simulink library "snn_champions_lib"  (R2026a)
settings: Solver=VariableStepAuto
(part 3 of 24)

== matlab function snn_champions_lib/Donatello_ACC_IIDM/SNN_ACC ==
  data: s input; accel output; v input; dv input; v_l input
function accel = SNN_ACC(s, v, dv, v_l)
%#codegen
% SP2 - campione Donatello + ACC-IIDM open-loop. ENTRAMBI in fixed -> HDL-ready.
%  Ingressi FIXED (>=20 bit frazionari); uscita accel (double). 1 cambio d'ingresso = 1
%  control-step = DT 0.1 s; ogni ingresso va tenuto >=341 campioni (time-mux).
  Tt = snn_types('fixed', 13);
  xn = local_normalize(s, v, dv, v_l, Tt);
  persistent pv xprev started acc
  if isempty(started)                % isempty(<persistent>) e' l'unica forma che il codegen
    pv = fi(zeros(5,1), 1, 21, 13);  % riconosce come prova di definizione: un test sul VALORE
    xprev = xn; started = true;      % fallirebbe con "undefined on some execution paths".
    Ta = acc_types('fixed'); acc = cast(0, 'like', Ta.out); go = true;
  else
    go = any(xn ~= xprev);           % edge-triggered: 1 campione = 1 inferenza
  end
  xprev = xn;
  [raw, valid] = snn_b2_fsm(xn, go);
  if valid
    pv = snn_decode_lut(raw, 64);
    % ⚠️ L'IIDM gira SOLO qui: una volta per control-step. A ogni clock vedrebbe Δv_l = 0 per
    %    340 campioni su 341 -> il filtro OU stimerebbe a_l ~ 0, in silenzio (spec §5).
    acc = acc_iidm_open(s, v, dv, v_l, pv(:), false, acc_types('fixed'));
  end
  accel = acc;                       % tenuto fino al control-step successivo
end

function xn = local_normalize(s, v, dv, v_l, T)
%LOCAL_NORMALIZE  fisico -> xn (fixed). Nel deployato la normalize gira in SW float e all'HDL
%  arriva gia' xn (HDL_PHASE §3.1); qui sta nel blocco per avere I/O fisico.
%  RECIPROCI a Q?.30 (NON Q?.20): verificato che con Q?.20 l'arrotondamento di xn devia di 1 LSB
%  dal path float ~1 volta su 25 step -> uno spike flippa -> i params divergono. Con Q?.30 e
%  ingressi con >=20 bit frazionari, xn e' IDENTICO al riferimento float (0 diff).
  invS   = fi(0.0066666666666666671, 1, 34, 30);
  invV   = fi(0.025000000000000001, 1, 34, 30);
  inv2DV = fi(0.025000000000000001, 1, 34, 30);
  invVL  = fi(0.025000000000000001, 1, 34, 30);
  DVc    = fi(20, 1, 24, 13);   % 24-13-1 = 10 bit interi: DV=20 ci sta
                                     % (con Q5.13/18bit saturerebbe a ~16 -> clamp sbagliato)
  d = dv;                            % clamp a +-DV. NB: d(:) = ... per NON cambiare il tipo di d
  if d >  DVc, d(:) =  DVc; end      %     (codegen: una variabile non puo' cambiare tipo, HDL_PHASE §9)
  if d < -DVc, d(:) = -DVc; end
  xn = cast(zeros(4,1), 'like', T.V);
  xn(1) = cast(s * invS, 'like', T.V);
  xn(2) = cast(v * invV, 'like', T.V);
  xn(3) = cast((d + DVc) * inv2DV, 'like', T.V);
  xn(4) = cast(v_l * invVL, 'like', T.V);
end

% ====================================================================================
% Funzioni locali INLINATE dai sorgenti veri (build_hdl_variants le legge a build-time).
% Le funzioni locali hanno precedenza sul path => il blocco e' SELF-CONTAINED.
% NON modificarle qui: si rigenerano con build_hdl_variants.
% ====================================================================================

function W = b2_rom_active() %#codegen
%B2_ROM_ACTIVE  Pesi del champion attivo (baked). GENERATO da gen_b2_rom('Donatello').
  W.fc = fi([1 1 -0.25 1;0.125 0.5 -0.0625 1;1 -1 1 0.125;1 0.125 0.5 -0.125;1 0.5 -0.0625 0.5;-0.0625 0.25 0 1;0 0.5 0.5 0.25;1 -0.25 2 -0.0625;1 0.125 -0.25 0.5;0.25 1 0.125 -0.25;0.25 -0.25 0.5 1;0.5 -0.5 0.5 0.25;1 0.25 -0.125 0.5;-1 1 0.25 0.5;1 0.5 1 -0.25;0.5 -0.25 0.5 0.0625;0.25 -0.25 1 -0.5;-0.5 -0.5 1 0.25;2 0 -0.25 0;-0.5 0.5 0.5 1;-0.125 -0.25 1 0;1 0.125 1 -0.5;-0.0625 1 0.5 0.125;1 1 -0.25 -0.125;2 0.5 0.5 -0.25;-0.125 0.5 0.25 -0.25;1 0.125 -0.0625 0.25;-0.5 -0.25 1 0.5;1 -0.125 0.125 0.5;1 -0.0625 0.5 0.25;1 0.5 1 0.125;0.125 0.25 0.5 0], 1, 16, 13);
  W.U = fi([0 0 -0.0625 -0.0625 -0.0625 0 0 0 -0.0625 0 0 0 0.0625 0 -0.125 0;-0.0625 0 -0.0625 0 0 0 0 0 0 0 -0.0625 0 0 0.0625 0 0;0.0625 -0.0625 -0.0625 0 -0.0625 -0.0625 0 0 0.0625 0 0.0625 0 0 0 0 0;0.0625 -0.0625 0 0 0 0 -0.0625 0 0 -0.0625 0.0625 -0.0625 0 -0.0625 0 -0.0625;0.0625 -0.0625 0 0 0 0 0.0625 0 0 0 0 -0.0625 0.0625 0 -0.0625 0;0 0.0625 0.0625 -0.0625 0.0625 0 0 0 0.0625 0.0625 0 0.0625 0 0 0 0;-0.0625 0.0625 0.0625 -0.0625 0 0 -0.0625 0.0625 0.0625 0.0625 0 0 -0.0625 0 0 0.0625;0 0 0.0625 0.0625 0 0 0 0 -0.0625 -0.0625 0 0 0 0 -0.0625 0;0 0 0 0 0.0625 -0.0625 0 0 -0.0625 -0.0625 -0.0625 0 0 0 0.0625 0;0 0 0 0 0.0625 0 0 0 0.0625 -0.0625 0 0.0625 0 0 0 0.0625;0 0 0 0 0 0 0 -0.0625 0 0 -0.0625 0 0 0 0 0.0625;0 0.0625 0 0.0625 0 0 0 0.0625 0 -0.0625 0 -0.0625 0.0625 0 0 0;-0.0625 0.0625 0 0 0 0 -0.0625 0 0.0625 0 -0.0625 0 0 0 0 0.125;0 0 0 0 0 0.0625 -0.0625 -0.0625 0 0.0625 0 0 0.0625 0.0625 0.0625 0;0.0625 0.0625 -0.0625 0 0 -0.0625 -0.0625 0 0 0 -0.0625 0 -0.0625 0 0 0;0.0625 0 0 0 -0.0625 -0.0625 -0.0625 0.0625 -0.0625 -0.0625 0 0.0625 0 0 0 0.0625;-0.0625 0 0 0 0.125 0.0625 -0.0625 -0.0625 0 0 0 0 -0.0625 0 -0.0625 0;0.0625 -0.0625 0 0.0625 0 -0.125 0 -0.0625 0 0 0.0625 -0.0625 0.0625 0 -0.0625 -0.0625;-0.0625 0 -0.0625 0.0625 -0.0625 0 -0.0625 0.0625 0.0625 -0.0625 0 0 -0.0625 0 0 -0.0625;0.0625 0.125 0 -0.0625 0 0 0 0 0.0625 0 0.0625 0.0625 0 0 -0.0625 0;0 -0.0625 0 0 -0.125 -0.0625 0 0.0625 -0.0625 -0.0625 0.0625 0 0.0625 -0.0625 -0.0625 -0.0625;0 0 0 0 -0.0625 0 0.0625 -0.0625 0 -0.0625 0.0625 0 0.0625 0 0 0;-0.0625 0.125 0 0 0 -0.0625 0 0 -0.0625 0.0625 0 0 0 0 0.0625 0;0 0 0 0 0 0 0 0 -0.0625 0 0.0625 0.125 0 0.0625 0 0.0625;0 -0.0625 0.0625 0 0 -0.0625 0 0 -0.0625 0 0 0.0625 0.0625 0 0 0;-0.0625 0 0 -0.125 0.0625 0.0625 0 0 0 0.0625 -0.0625 0.0625 -0.0625 0.0625 0.0625 0;0.0625 -0.0625 0 0 0 0 0.0625 0 -0.0625 0 0 0 0 0 0 0.0625;0 0 0 0.125 0 0 0 0.0625 -0.0625 0 0.0625 -0.0625 0 0.0625 0 0;0 0.0625 0.0625 0 0 0.0625 -0.0625 0 0 0.0625 0 0 -0.0625 0 0.0625 0.125;0 0.0625 0.0625 0.0625 0.0625 0.0625 0 0 0 0.0625 -0.0625 0.0625 -0.0625 0 0 0;0 0 0.0625 0 0 0.0625 -0.0625 -0.0625 0.0625 0.0625 -0.0625 0.125 0.0625 0 0 0;0 0 -0.0625 0.0625 0.0625 0 0 0.125 0 0.0625 0.0625 0.0625 0 -0.0625 0.0625 0], 1, 16, 13);
  W.Vr = fi([0 -0.125 -0.0625 -0.0625 0 0 -0.0625 -0.0625 0 -0.0625 -0.0625 0 0 0 -0.0625 -0.0625 0 0 0.0625 0 0 -0.125 0 0.0625 0 0 -0.0625 0 0 0 0 0;0.0625 0.0625 0 0 0 0 0.0625 0 0 0.0625 0.0625 0 0 0 0 0.0625 0 -0.0625 0 0.0625 0 0 0.0625 0 0.0625 0 0 0.125 -0.0625 0.125 0 0;0 0.0625 0 0.0625 0 0 -0.0625 0 0 0 0 0 0 0.0625 0 0 0.0625 0 0.0625 0 0 0.0625 0.0625 0 -0.0625 -0.0625 0 0 0 0.0625 0 0.0625;0 -0.0625 -0.0625 0 0 0 0 -0.0625 0 0 0.0625 0.0625 0 0 0 0.0625 0.0625 0 -0.0625 -0.0625 -0.0625 -0.0625 0.0625 0 0 0 0 0 0.0625 -0.0625 -0.0625 0;0 0 0.0625 0 -0.0625 0.0625 0.0625 0.0625 0 0 0.0625 0 0.0625 0.0625 0.0625 0 0.0625 0 0.0625 0 0.0625 0 0 0.0625 0.0625 0 0.125 0 0 0.0625 0.0625 0;0 0.0625 -0.125 0 0 0 0 0 0 -0.0625 -0.0625 0 0 0.0625 0.125 0.0625 0 0.0625 -0.0625 0.0625 0.0625 0 0.0625 -0.0625 0 -0.0625 0 0 0 0.0625 0 0;0 -0.0625 -0.0625 0 0 -0.0625 0 -0.0625 0 0 -0.0625 -0.0625 -0.0625 0.0625 -0.0625 0 0 -0.0625 0.0625 -0.125 -0.0625 0 -0.0625 -0.0625 -0.0625 0 0 -0.125 -0.0625 0 0 -0.0625;0 0 -0.0625 -0.0625 0.0625 0 -0.0625 0 -0.0625 0 0.0625 -0.0625 0.0625 0.0625 0.0625 0 0 0 0 -0.0625 0 -0.0625 0 0 0 0 -0.0625 -0.0625 0 0 0 0;-0.0625 0.0625 0 0.0625 0 0.0625 -0.0625 0 0.0625 0 0.0625 0 0 0.0625 0 0 0 0 0.0625 -0.0625 0.0625 0 0.0625 0 0 0.125 0.0625 0.0625 0.0625 0.0625 0 0;0.0625 0.0625 0 0.0625 0.0625 0.0625 0.0625 0.0625 0.0625 0 0.0625 0 0.0625 0.0625 0 -0.0625 0.0625 0 0.0625 0.0625 0 0.0625 0.0625 0 0.0625 0.0625 0 0 0 0 0 0;0 -0.0625 -0.0625 0 -0.0625 0 0 0 0 0 -0.0625 -0.125 -0.0625 -0.0625 0 -0.0625 -0.0625 0 0 -0.0625 -0.0625 0 0 0 0 -0.0625 0 -0.0625 0 0 -0.0625 0;0 0 0 0.0625 0 0 0.0625 0 0 0 0 0 0.0625 0 0 0.125 -0.0625 0 0.0625 0.0625 0 0 0.0625 0.0625 0 0.0625 0.0625 0 0 0 0 0;-0.0625 0 0 0 0.0625 0.0625 0 -0.0625 -0.0625 -0.0625 -0.0625 0 0 -0.0625 0 -0.0625 0 0 0 -0.0625 0 -0.0625 0 0 -0.0625 -0.0625 0 0 -0.0625 0 0.0625 0;0.0625 0 0 0.0625 0 0 0 -0.0625 0 0.0625 0 -0.0625 0 0.0625 0.0625 0 0.0625 0.0625 0 0.0625 0 0 0 0.0625 0.0625 0 0 0.125 0 0 0.0625 -0.0625;0.0625 0 0 0.0625 0 0.0625 0 0 0 0.0625 -0.0625 -0.0625 0 0.125 0 0 0 0 -0.0625 0 0.0625 0 0.0625 -0.0625 0.0625 0 0 0 0 0 0.0625 0;0 0 0 0.0625 0 0.0625 0 0.0625 0 0 0.0625 0.0625 0 0 0 0.0625 -0.0625 0 0.0625 0.0625 0.0625 0 0 0.0625 0.125 0 0 0 0 0 0.0625 0], 1, 19, 13);
  W.Wout = fi([-0.25 -0.125 -0.0625 -0.25 -0.25 0.25 0.25 -0.5 0.125 0.125 0.5 0.25 0.5 -0.125 0.25 0.25 -0.5 -0.25 0.0625 0.25 -0.25 0.0625 0 0.125 -0.25 0.25 0.25 -0.25 0 0 0.125 0.5;0.125 -0.125 0.25 -0.25 -0.125 0 -0.25 0 -0.25 0 0 0 -0.5 -0.5 0.125 0.25 -0.5 0.125 -0.25 0 0.25 0.25 -0.25 0.25 0.25 0 0.5 -0.25 -0.125 -0.25 0.0625 0.0625;0 -0.25 -0.25 0.125 -0.5 -0.0625 0 -0.125 0.125 0 0.25 -0.0625 -0.25 0.25 0.0625 -0.125 -0.25 0.125 -0.5 0.125 0.25 -0.5 -0.25 -0.25 0.25 0.25 0 0.5 -0.125 -0.5 0.125 0.125;0.5 0 0.25 0.25 0.25 -0.5 0.25 -0.25 0.5 0 -0.5 0.125 -0.0625 -0.5 -0.125 0.0625 0.25 -0.125 0.25 0.0625 0 0.0625 -0.25 -0.25 -0.125 -0.5 -0.25 0 -0.25 -0.125 -0.0625 -0.0625;-0.25 0 -0.0625 0.0625 0 -0.25 -0.125 -0.0625 -0.25 0 -0.0625 0.125 0.0625 0.25 -0.0625 -0.25 0.125 -0.25 -0.0625 -0.125 -0.25 -0.125 0.25 0.25 0.0625 0.25 -0.5 0.0625 0.25 0.25 -0.25 0.125], 1, 16, 13);
  W.bth = fi([1.4830578565597534;1.4914478063583374;1.4758200645446777;1.4738426208496094;1.4738566875457764;1.5251744985580444;1.5266332626342773;1.4767427444458008;1.4758551120758057;1.5250141620635986;1.5258395671844482;1.5129754543304443;1.5257152318954468;1.5249043703079224;1.5155367851257324;1.5183815956115723;1.5177655220031738;1.4894863367080688;1.4749715328216553;1.5253423452377319;1.4770052433013916;1.4827579259872437;1.5239431858062744;1.5230189561843872;1.4776254892349243;1.5125672817230225;1.5243701934814453;1.4934873580932617;1.5239229202270508;1.5202276706695557;1.5248651504516602;1.5149734020233154], 1, 19, 13);
  W.tj = fi([0.49987733364105225;0.49987733364105225;0.49987733364105225;0.49987733364105225;0.49987733364105225;0.49987733364105225;0.49987733364105225;0.49987733364105225;0.49987733364105225;0.49987733364105225;0.49987733364105225;0.49987733364105225;0.49987733364105225;0.49987733364105225;0.49987733364105225;0.49987733364105225;0.49987733364105225;0.49987733364105225;0.49987733364105225;0.49987733364105225;0.49987733364105225;0.49987733364105225;0.49987733364105225;0.49987733364105225;0.49987733364105225;0.49987733364105225;0.49987733364105225;0.49987733364105225;0.49987733364105225;0.49987733364105225;0.49987733364105225;0.49987733364105225], 1, 19, 13);
  W.delays = [3 5 1 2;2 4 4 4;2 4 0 4;5 0 5 5;1 2 2 2;4 1 4 2;0 4 0 1;0 1 0 1;2 2 1 3;1 2 5 2;0 5 1 2;0 5 3 1;2 0 0 4;2 2 3 4;4 4 5 0;4 5 0 2;0 4 4 3;5 5 4 2;4 5 4 2;3 0 3 1;3 2 0 4;0 4 2 0;5 4 5 2;4 4 3 3;5 3 4 5;2 2 3 1;3 3 5 3;1 3 0 3;1 0 3 2;2 3 4 4;2 4 5 0;1 2 4 0];
  W.sh = 3;
  W.invS = fi(0.0066666666666666671, 1, 24, 20);
  W.invV = fi(0.025000000000000001, 1, 24, 20);
  W.invVL = fi(0.025000000000000001, 1, 24, 20);
  W.inv2DV = fi(0.025000000000000001, 1, 24, 20);
  W.DV = fi(20, 1, 20, 13);
end


function T = snn_types(dt, nfrac)
%SNN_TYPES Prototipi di tipo per il core type-parametrizzato.
%  dt = 'double' (parita' vs golden) | 'fixed' (HDL, Qm.n).
%  nfrac (opz., default 5) = bit frazionari del path fixed; i bit INTERI restano
%  fissi (range invariato), varia solo la risoluzione -> per tarare i word-length
%  col ginocchio errore/risorse (run_fixed_sweep). nfrac=5 == config storica.
  if nargin < 2, nfrac = 5; end
  switch dt
    case 'double'
      z = double([]);
      T = struct('V', z, 'fatigue', z, 'acc', z, 'accw', z, 'raw', z, 'w', z);
    case 'fixed'
      f = nfrac;
      T = struct( ...
        'V',       fi([], true, 6 + f, f), ...    % Q5.f  (int 5)
        'fatigue', fi([], true, 4 + f, f), ...    % Q3.f  (int 3)
        'acc',     fi([], true, 6 + f, f), ...    % accumulatore I_input Q5.f (int 5: un tap di delay arriva a ~8)
        'accw',    fi([], true, 13 + f, f + 4), ...% accumulatore LARGO Q8.(f+4): +4 frac per shift po2 esatti
        'raw',     fi([], true, 8 + f, f), ...    % readout LI Q7.f (int 7)
        'w',       fi([], true, 3 + f, f));       % pesi po2 Q2.f (esatti per f>=5)
    otherwise
      error('snn_types:dt', 'dt deve essere ''double'' o ''fixed''');
  end
end


function [raw, valid] = snn_b2_fsm(xn, start) %#codegen
%SNN_B2_FSM  [B2] SNN Donatello time-multiplexato (1 neurone/clock) con hdl.RAM.
%  Mirror BIT-EXACT dell'aritmetica di snn_core, serializzato: V/fatigue in hdl.RAM,
%  pesi in ROM (coder.const), pipeline a 2 stadi per la latenza RAM (read->compute->write,
%  1 sola chiamata RAM/ciclo). Streaming: start=1 -> nuova control-step; valid=1 -> raw pronto.
  W = coder.const(b2_rom_active());
  T = snn_types('fixed', 13);
  hidden = 32; nt = 10; rnk = coder.const(size(W.U, 2)); out = 5; sh = W.sh;

  persistent Vram fatram xbuf xnreg t_lr t_lr_nxt V_LI wacc ...
             tickc rc written phase ...
             pR_valid pR_idx pCx_valid pCx_idx pCx_xsel pCx_Vread pCx_fat ...
             pCm_valid pCm_idx pCm_Iip pCm_recip pCm_Vread pCm_fat ...
             pCa_valid pCa_idx pCa_reci pCa_Ii pCa_Vread pCa_fat ...
             pC1_valid pC1_idx pC1_Ii pC1_reci pC1_Vread pC1_fat ...
             pC2i_valid pC2i_idx pC2i_Vi pC2i_eth pC2i_fat ...
             pC2a_valid pC2a_idx pC2a_nCV pC2a_sib pC2a_fat ...
             pC_valid pC_idx pC_V pC_fat rawreg inited
  if isempty(inited)
    Vram   = hdl.RAM('RAMType', 'Dual port');
    fatram = hdl.RAM('RAMType', 'Dual port');
    xbuf   = cast(zeros(4, 6), 'like', T.V);
    xnreg  = cast(zeros(4, 1), 'like', T.V);
    t_lr     = cast(zeros(rnk, 1), 'like', T.acc);
    t_lr_nxt = cast(zeros(rnk, 1), 'like', T.acc);
    V_LI = cast(zeros(out, 1), 'like', T.raw);
    wacc = cast(zeros(out, 1), 'like', T.raw);
    tickc = uint8(0); rc = uint8(0); written = uint8(0); phase = uint8(0);
    pR_valid = false; pR_idx = uint8(0);
    pCx_valid = false; pCx_idx = uint8(0);
    pCx_xsel = cast(zeros(4, 1), 'like', T.V);
    pCx_Vread = cast(0, 'like', T.V); pCx_fat = cast(0, 'like', T.fatigue);
    pCm_valid = false; pCm_idx = uint8(0);
    pCm_Iip = cast(zeros(4, 1), 'like', T.accw); pCm_recip = cast(zeros(rnk, 1), 'like', T.accw);
    pCm_Vread = cast(0, 'like', T.V); pCm_fat = cast(0, 'like', T.fatigue);
    pCa_valid = false; pCa_idx = uint8(0);
    pCa_reci = cast(zeros(rnk/4, 1), 'like', T.accw);   % rnk/4 somme parziali (dopo 2 livelli d'albero)
    pCa_Ii = cast(0, 'like', T.accw);
    pCa_Vread = cast(0, 'like', T.V); pCa_fat = cast(0, 'like', T.fatigue);
    pC1_valid = false; pC1_idx = uint8(0);
    pC1_Ii = cast(0, 'like', T.accw); pC1_reci = cast(0, 'like', T.accw);
    pC1_Vread = cast(0, 'like', T.V); pC1_fat = cast(0, 'like', T.fatigue);
    % [2d R8] prototipi dei tipi LARGHI di Vi/eth (l'addizione fixed li allarga oltre T.V): servono per
    % registrarli fra C2i (Vi/eth) e C2a (soglia/nC_V) senza conflitto di tipo in codegen.
    zV = cast(0, 'like', T.V); zA = cast(0, 'like', T.accw); zF = cast(0, 'like', T.fatigue);
    Vi0  = cast(zV - bitsra(zV, sh), 'like', T.V) + (zA + zA);
    eth0 = cast(zV, 'like', T.V) + cast(max(zF, zF), 'like', T.V);
    pC2i_valid = false; pC2i_idx = uint8(0);
    pC2i_Vi = cast(0, 'like', Vi0); pC2i_eth = cast(0, 'like', eth0);
    pC2i_fat = cast(0, 'like', T.fatigue);
    pC2a_valid = false; pC2a_idx = uint8(0);
    pC2a_nCV = cast(0, 'like', T.V); pC2a_sib = cast(0, 'like', T.V);
    pC2a_fat = cast(0, 'like', T.fatigue);
    pC_valid = false; pC_idx = uint8(0);
    pC_V = cast(0, 'like', T.V); pC_fat = cast(0, 'like', T.fatigue);
    rawreg = cast(zeros(out, 1), 'like', T.raw);
    inited = true;
  end

  valid = false;
  raw = rawreg;

  % ---------- helper x_buf: shift + inserimento xnreg (inizio tick) ----------
  % (fatto inline dove serve)

  if phase == uint8(0)
    % IDLE: su start latcha xn, fa lo shift del tick 0, avvia la pipeline
    if start
      xnreg = xn;
      xbuf(:, 2:6) = xbuf(:, 1:5); xbuf(:, 1) = xnreg;   % tick 0 shift+insert
      tickc = uint8(0); rc = uint8(0); written = uint8(0);
      wacc = cast(zeros(out, 1), 'like', T.raw);
      pR_valid = false; pC_valid = false;
      phase = uint8(1);
    end
    % passo RAM idle (mantiene coerenza)
    [~, ~] = Vram(cast(0,'like',T.V), uint8(0), false, uint8(0));
    [~, ~] = fatram(cast(0,'like',T.fatigue), uint8(0), false, uint8(0));
    return;
  end

  % ---------- FASE 1: RUN (pipeline 2-stadi, 1 chiamata RAM/ciclo) ----------
  % indirizzo di lettura per questo ciclo (neurone rc, se ancora da leggere)
  if rc < uint8(hidden), rdAddr = rc; else, rdAddr = uint8(0); end

  % UNA chiamata RAM: scrive il risultato dello stadio C (pC), legge rdAddr
  [~, Vread]   = Vram(pC_V,   pC_idx, pC_valid, rdAddr);
  [~, fatread] = fatram(pC_fat, pC_idx, pC_valid, rdAddr);
  if pC_valid
    written = written + uint8(1);
  end

  % --- STADIO Cx (mux xbuf: seleziona i 4 ingressi ritardati): dal neurone pR ---
  % [2d R9] separo il mux a indice variabile xbuf(j,col) dal DSP mult: Cx registra i 4 valori selezionati
  % (xsel), Cm fa solo i moltiplicatori dai valori registrati -> il mult (~4,6ns) resta l'unico op del suo path.
  nCx_valid = false; nCx_idx = uint8(0);
  nCx_xsel = cast(zeros(4, 1), 'like', T.V);
  nCx_Vread = cast(0, 'like', T.V); nCx_fat = cast(0, 'like', T.fatigue);
  if pR_valid
    i = double(pR_idx) + 1;
    for j = 1:4
      col = double(W.delays(i, j)) + 1;
      nCx_xsel(j) = xbuf(j, col);
    end
    nCx_Vread = Vread; nCx_fat = fatread;
    nCx_valid = true; nCx_idx = pR_idx;
  end

  % --- STADIO Cm (MAC: 16 prodotti reci + 4 prodotti Ii, REGISTRATI): dagli ingressi mux registrati pCx ---
  % [2d R6] isolo i moltiplicatori: Cm calcola e REGISTRA i prodotti (uscite DSP), Ca fa gli alberi dai
  % prodotti registrati -> il DSP mult (~4,6ns) esce dal path degli alberi (mappato sul registro P del DSP48).
  % Bit-exact: stessi prodotti, solo registrati.
  nCm_valid = false; nCm_idx = uint8(0);
  nCm_Iip = cast(zeros(4, 1), 'like', T.accw);
  nCm_recip = cast(zeros(rnk, 1), 'like', T.accw);
  nCm_Vread = cast(0, 'like', T.V); nCm_fat = cast(0, 'like', T.fatigue);
  if pCx_valid
    i = double(pCx_idx) + 1;
    for j = 1:4
      nCm_Iip(j) = cast(cast(W.fc(i, j), 'like', T.w) * pCx_xsel(j), 'like', T.accw);
    end
    for r = 1:rnk
      nCm_recip(r) = cast(cast(W.U(i, r), 'like', T.w) * t_lr(r), 'like', T.accw);
    end
    nCm_Vread = pCx_Vread; nCm_fat = pCx_fat;
    nCm_valid = true; nCm_idx = pCx_idx;
  end

  % --- STADIO Ca (alberi: Ii 4->1, reci L1-L2 16->4): dai prodotti registrati pCm ---
  kmid = coder.const(rnk / 4);                    % rnk=16 -> 4 parziali dopo 2 livelli
  nCa_valid = false; nCa_idx = uint8(0);
  nCa_reci = cast(zeros(kmid, 1), 'like', T.accw);
  nCa_Ii = cast(0, 'like', T.accw);
  nCa_Vread = cast(0, 'like', T.V); nCa_fat = cast(0, 'like', T.fatigue);
  if pCm_valid
    % Ii ad albero (4->2->1) dai prodotti registrati
    Ii_p = pCm_Iip;
    Ii_p(1) = cast(Ii_p(1) + Ii_p(2), 'like', T.accw);
    Ii_p(2) = cast(Ii_p(3) + Ii_p(4), 'like', T.accw);
    nCa_Ii  = cast(Ii_p(1) + Ii_p(2), 'like', T.accw);
    % reci: primi 2 livelli d'albero (16->4) dai prodotti registrati
    reci_p = pCm_recip;
    lvsz_a = coder.const(round(rnk ./ 2 .^ (1:2)));   % rnk=16 -> [8 4]
    for lev = 1:2
      for q = 1:lvsz_a(lev)
        reci_p(q) = cast(reci_p(2*q - 1) + reci_p(2*q), 'like', T.accw);
      end
    end
    nCa_reci = reci_p(1:kmid);            % rnk/4 somme parziali (T.accw)
    nCa_Vread = pCm_Vread; nCa_fat = pCm_fat;
    nCa_valid = true; nCa_idx = pCm_idx;
  end

  % --- STADIO C1 (SECONDA meta' dell'albero reci): dal registro pCa ---
  nC1_valid = false; nC1_idx = uint8(0);
  nC1_Ii = cast(0, 'like', T.accw); nC1_reci = cast(0, 'like', T.accw);
  nC1_Vread = cast(0, 'like', T.V); nC1_fat = cast(0, 'like', T.fatigue);
  if pCa_valid
    reci_p2 = pCa_reci;                  % kmid parziali
    lvsz_b = coder.const(round(kmid ./ 2 .^ (1:log2(kmid))));   % kmid=4 -> [2 1]
    for lev = 1:numel(lvsz_b)
      for q = 1:lvsz_b(lev)
        reci_p2(q) = cast(reci_p2(2*q - 1) + reci_p2(2*q), 'like', T.accw);
      end
    end
    nC1_reci = reci_p2(1);
    nC1_Ii = pCa_Ii; nC1_Vread = pCa_Vread; nC1_fat = pCa_fat;   % Vi/soglia -> C2 (tipi larghi restano locali)
    nC1_valid = true; nC1_idx = pCa_idx;
  end

  % --- STADIO C2i (calcola Vi ed eth, tipi larghi 28-bit): dal registro pC1 ---
  % [2d R8] separo Vi/eth (catena di add 28-bit, era il collo in C2a-R7) dalla soglia/nC_V: C2i li produce
  % e REGISTRA (tipi larghi via prototipo Vi0/eth0 in init; init nel corpo via 'like' pC2i_*). Bit-exact.
  nC2i_valid = false; nC2i_idx = uint8(0);
  nC2i_Vi = cast(0, 'like', pC2i_Vi); nC2i_eth = cast(0, 'like', pC2i_eth);
  nC2i_fat = cast(0, 'like', T.fatigue);
  if pC1_valid
    i2 = double(pC1_idx) + 1;
    nC2i_Vi  = cast(pC1_Vread - bitsra(pC1_Vread, sh), 'like', T.V) + (pC1_Ii + pC1_reci);
    nC2i_eth = cast(W.bth(i2), 'like', T.V) + cast(max(pC1_fat, cast(0,'like',T.fatigue)), 'like', T.V);
    nC2i_fat = pC1_fat;
    nC2i_valid = true; nC2i_idx = pC1_idx;
  end

  % --- STADIO C2a (soglia + nC_V + accumulo readout): dal registro pC2i ---
  nC2a_valid = false; nC2a_idx = uint8(0);
  nC2a_nCV = cast(0, 'like', T.V); nC2a_sib = cast(0, 'like', T.V);
  nC2a_fat = cast(0, 'like', T.fatigue);
  if pC2i_valid
    i2  = double(pC2i_idx) + 1;
    si  = pC2i_Vi >= pC2i_eth;
    sib = cast(si, 'like', T.V);
    nC2a_nCV = cast(pC2i_Vi - sib * pC2i_eth, 'like', T.V);
    nC2a_sib = sib; nC2a_fat = pC2i_fat;
    nC2a_valid = true; nC2a_idx = pC2i_idx;
    if si
      for o = 1:out
        wacc(o) = cast(wacc(o) + W.Wout(o, i2), 'like', T.raw);
      end
      for r = 1:rnk
        t_lr_nxt(r) = cast(t_lr_nxt(r) + cast(W.Vr(r, i2), 'like', T.acc), 'like', T.acc);
      end
    end
  end

  % --- STADIO C2b (nC_fat = leaky(fat) + sib*tj): dal registro pC2a; nC_V passa attraverso ---
  nC_valid = false; nC_idx = uint8(0);
  nC_V = cast(0, 'like', T.V); nC_fat = cast(0, 'like', T.fatigue);
  if pC2a_valid
    i3 = double(pC2a_idx) + 1;
    nC_fat = cast(cast(pC2a_fat - bitsra(pC2a_fat, sh), 'like', T.fatigue) + pC2a_sib * cast(W.tj(i3), 'like', T.V), 'like', T.fatigue);
    nC_V   = pC2a_nCV;
    nC_valid = true; nC_idx = pC2a_idx;
  end

  % --- STADIO R (read schedule): programma la lettura del neurone rc ---
  nR_valid = false; nR_idx = uint8(0);
  if rc < uint8(hidden)
    nR_valid = true; nR_idx = rc;
    rc = rc + uint8(1);
  end

  % avanza i registri pipeline (R -> Cm -> Ca -> C1 -> C2 -> write)
  pR_valid = nR_valid; pR_idx = nR_idx;
  pCx_valid = nCx_valid; pCx_idx = nCx_idx; pCx_xsel = nCx_xsel; pCx_Vread = nCx_Vread; pCx_fat = nCx_fat;
  pCm_valid = nCm_valid; pCm_idx = nCm_idx; pCm_Iip = nCm_Iip; pCm_recip = nCm_recip; pCm_Vread = nCm_Vread; pCm_fat = nCm_fat;
  pCa_valid = nCa_valid; pCa_idx = nCa_idx; pCa_reci = nCa_reci; pCa_Ii = nCa_Ii; pCa_Vread = nCa_Vread; pCa_fat = nCa_fat;
  pC1_valid = nC1_valid; pC1_idx = nC1_idx; pC1_Ii = nC1_Ii; pC1_reci = nC1_reci; pC1_Vread = nC1_Vread; pC1_fat = nC1_fat;
  pC2i_valid = nC2i_valid; pC2i_idx = nC2i_idx; pC2i_Vi = nC2i_Vi; pC2i_eth = nC2i_eth; pC2i_fat = nC2i_fat;
  pC2a_valid = nC2a_valid; pC2a_idx = nC2a_idx; pC2a_nCV = nC2a_nCV; pC2a_sib = nC2a_sib; pC2a_fat = nC2a_fat;
  pC_valid = nC_valid; pC_idx = nC_idx; pC_V = nC_V; pC_fat = nC_fat;

  % --- fine tick: tutti i 32 neuroni scritti ---
  if written >= uint8(hidden)
    V_LI = cast(cast(V_LI - bitsra(V_LI, 3), 'like', T.raw) + wacc, 'like', T.raw);
    wacc = cast(zeros(out, 1), 'like', T.raw);
    t_lr = t_lr_nxt;
    t_lr_nxt = cast(zeros(rnk, 1), 'like', T.acc);
    written = uint8(0); rc = uint8(0);
    pR_valid = false; pCx_valid = false; pCm_valid = false; pCa_valid = false; pC1_valid = false; pC2i_valid = false; pC2a_valid = false; pC_valid = false;
    if tickc >= uint8(nt - 1)
      rawreg = V_LI; raw = V_LI; valid = true;
      phase = uint8(0); tickc = uint8(0);
    else
      tickc = tickc + uint8(1);
      xbuf(:, 2:6) = xbuf(:, 1:5); xbuf(:, 1) = xnreg;   % shift+insert per il tick successivo
    end
  end
end

% ---- ROM pesi del champion attivo: in b2_rom_active.m (baked, GENERATO da gen_b2_rom(name)) ----


function p = snn_decode_lut(raw, N) %#codegen
%SNN_DECODE_LUT  Decode Donatello con sigmoide via LUT a N punti su [-8,8) + interp lineare.
%  Generalizza snn_decode_hdl (N=256). N = coder.const, potenza di 2 (scala indice = N/16).
%  Costanti Donatello baked (lo sweep e' Donatello-only). Bit-identico a snn_decode_hdl per N=256.
%
%  ⚠️ SINGLE SOURCE (R4, 2026-07-19): il corpo e' ora la composizione di decode_a + decode_b, che sono
%  le DUE FASI che la chart esegue in due clock distinti -- il decode era il collo (pv_3, 31 livelli:
%  quattro moltiplicatori in serie piu' la lettura di tabella, tutto in un clock).
%  Composte qui in una chiamata sola perche' (a) i chiamanti non cambiano (snn_top_b2, le varianti
%  Donatello_LUT16..512) e (b) i cancelli provano ESATTAMENTE il codice che gira in hardware, non un
%  suo gemello. Il taglio e' fra `frac` e la lettura di `sgtab`: espressioni invariate, solo separate.
  [k, frac] = decode_a(raw, N);
  sv        = decode_b(k, frac, N);
  p         = decode_c(sv);   % [R10] scalatura finale in una fase a se'
end


function [k, frac] = decode_a(raw, N) %#codegen
%DECODE_A  [R4/R12] Prima meta' del decode: dal readout grezzo all'INDICE di tabella + frazione.
%
%  ⚠️ SINGLE SOURCE: composizione di decode_a1 (normalizzazione) e decode_a2 (scala/indice/frazione),
%  che la chart esegue in DUE clock -- i due moltiplicatori erano in serie (collo a 57,5 MHz).
%  Composta qui per i chiamanti funzionali (snn_decode_lut) e perche' i cancelli provino il codice vero.
%
%  ⚠️ NON si time-multiplexano i 5 parametri (restano srotolati): sarebbe un'ottimizzazione di AREA, e
%  di area ce n'e' in abbondanza. Serve solo profondita'.
  adjv        = decode_a1(raw);
  [k, frac]   = decode_a2(adjv, N);
end


function adjv = decode_a1(raw) %#codegen
%DECODE_A1  [R12] Prima parte del decode: normalizzazione (raw - offset)*invtau.
%  Separata da decode_a2 perche' i due moltiplicatori (invtau e scale) erano in serie nello stesso
%  clock -- era il collo a 57,5 MHz (dfrv, 18 livelli). `adj` ha il tipo Tadj GIA' DICHIARATO
%  nell'originale, quindi qui non si stringe nulla (nessun rischio §2.1).
%  Espressione VERBATIM da snn_decode_lut.
  Traw  = numerictype(1,21,13); Tadj = numerictype(1,18,13); Titau = numerictype(1,18,16);
  offset = coder.const(fi([-0.40404 -0.39012 1.7718 2.6884 -0.95578].', Traw));
  invtau = coder.const(fi([0.1 1/3 0.1 1/3 1/3].', Titau));
  adjv = fi(zeros(5,1), Tadj);
  for i = 1:5
    adjv(i) = fi((raw(i) - offset(i)) * invtau(i), Tadj);
  end
end


function [k, frac] = decode_a2(adjv, N) %#codegen
%DECODE_A2  [R12] Seconda parte: scala su [0,N), indice di tabella e frazione.
%  Espressioni VERBATIM da snn_decode_lut, con `adj` gia' calcolato da decode_a1.
  Tadj = numerictype(1,18,13); Ts = numerictype(1,16,14); Tsc = numerictype(0,23,13);
  scale = coder.const(N / 16);                                    % punti per unita' su [-8,8)
  Tsm   = numerictype(0, 8, 0);                                   % moltiplicatore scala (<=32)
  k    = zeros(5, 1, 'int32');
  frac = fi(zeros(5,1), Ts);
  for i = 1:5
    scaled = fi((adjv(i) + fi(8, Tadj)) * fi(scale, Tsm), Tsc);    % (adj+8)*scale in [0,N)
    ki = int32(floor(scaled));
    if ki < int32(0),     ki = int32(0);     end
    if ki > int32(N - 2), ki = int32(N - 2); end
    k(i)    = ki;
    frac(i) = fi(scaled - fi(double(ki), Tsc), Ts);
  end
end


function sv = decode_b(k, frac, N) %#codegen
%DECODE_B  [R4/R10/R17] Seconda fase del decode: tabella + interpolazione lineare -> s.
%  ⚠️ SINGLE SOURCE: composizione di decode_b1 (letture + differenza) e decode_b2 (interpolazione), che
%  la chart esegue in DUE clock. Composta qui per i chiamanti funzionali e per i cancelli.
  [s0v, delv] = decode_b1(k, N);
  sv          = decode_b2(s0v, delv, frac);
end


function [s0v, delv] = decode_b1(k, N) %#codegen
%DECODE_B1  [R17] Letture della tabella + differenza: s0 = sgtab(k), del = sgtab(k+1) - sgtab(k).
%  Separata da decode_b2 perche' letture, sottrazione, moltiplicazione e somma erano tutte nello stesso
%  clock -- era il collo a 77,6 MHz (dsv, 14 livelli). Espressioni VERBATIM da snn_decode_lut.
  Ts    = numerictype(1,16,14);
  scale = coder.const(N / 16);
  sgtab = coder.const(fi(1 ./ (1 + exp(-(-8 + (0:N-1) / scale))), Ts));  % 1xN
  s0v  = fi(zeros(5,1), Ts);
  delv = fi(zeros(5,1), Ts);
  for i = 1:5
    s0 = sgtab(k(i) + 1); s1 = sgtab(k(i) + 2);
    s0v(i)  = s0;
    delv(i) = fi(s1 - s0, Ts);
  end
end


function sv = decode_b2(s0v, delv, frac) %#codegen
%DECODE_B2  [R17] Interpolazione lineare: s = s0 + frac*del. Espressione VERBATIM da snn_decode_lut.
  Ts = numerictype(1,16,14);
  sv = fi(zeros(5,1), Ts);
  for i = 1:5
    sv(i) = fi(s0v(i) + frac(i) * delv(i), Ts);
  end
end


function p = decode_c(sv) %#codegen
%DECODE_C  Scalatura finale -> i 5 parametri. [R10] fase a se' nel controllore.
%  [A3] Ora e' la COMPOSIZIONE di decode_c1 (i prodotti, a precisione piena) + decode_c2 (somma
%  dell'offset + cast). Composta qui perche' (a) i chiamanti non cambiano e (b) i cancelli provano
%  ESATTAMENTE il codice che gira in hardware, non un suo gemello.
%  La chart nella variante `p6` chiama le due meta' in due fasi distinte: e' li' che il taglio serve,
%  perche' separa i DSP dalla catena di CARRY4 che domina il path critico.
  pr = decode_c1(sv);
  p  = decode_c2(pr);
end


function pr = decode_c1(sv) %#codegen
%DECODE_C1  [A3] Prima meta' di decode_c: i SOLI PRODOTTI hilo.*sv.
%  Taglio dentro l'operazione, non fra le operazioni: il collo di Donatello e' `lo + hilo*sv`, dove i
%  DSP fanno la moltiplicazione ma la somma finisce in fabric come catena di 15 CARRY4 in serie
%  (misurato: 24,307 ns = logica 15,490 + routing 8,817, 23 livelli).
%  Registrare il prodotto separa DSP e addizionatore in due clock.
%
%  ⚠️ LARGHEZZA PIENA: il prodotto NON va stretto qui. Stringere un parziale prima dell'uso e' il bug
%  §2.1 di questo progetto — cambierebbe la matematica. Il tipo si lascia DEDURRE dall'espressione.
  Tp   = numerictype(1,21,13);
  hilo = coder.const(fi([37 2 4 2.2 2.5].', Tp));
  pr   = hilo .* sv;                  % tipo dedotto = precisione piena
end


function p = decode_c2(pr) %#codegen
%DECODE_C2  [A3] Seconda meta' di decode_c: somma dell'offset + cast finale ai 5 parametri.
%  Riceve il prodotto a PRECISIONE PIENA da decode_c1 (registrato) e fa `lo + pr`, poi il cast a Q8.13.
%  Aritmetica IDENTICA a decode_c: stesso ordine, stesso singolo cast finale -> bit-exact per
%  costruzione. Ma "per costruzione" non e' un cancello: lo prova run_block_traj_test (dmax=0).
  Tp = numerictype(1,21,13);
  lo = coder.const(fi([8 0.5 1 0.3 0.5].', Tp));
  p  = fi(zeros(5,1), Tp);
  for i = 1:5
    p(i) = fi(lo(i) + pr(i), Tp);
  end
end


function [accel, pairs] = acc_iidm_open(s, v, dv, v_l, p, rst, T) %#codegen
%ACC_IIDM_OPEN  ACC-IIDM **open-loop**: accel = f(stato, parametri). NON integra v ne' s.
%  s, v, dv, v_l : stato fornito DA FUORI (il loop lo chiude il sistema che testa)
%  p             : [v0; T; s0; a; b]
%  rst           : true -> azzera lo stato del filtro OU (inizio di una nuova traiettoria)
%  T (opz.)      : prototipi di tipo (acc_types). Assente/vuoto -> DOUBLE (riferimento + plant
%                  cf_plant_lib/ACC_IIDM); popolato -> FIXED (blocco HDL-ready Donatello_ACC_IIDM).
%                  Type-parametrico come snn_core: UNICA fonte, perche' due implementazioni della
%                  stessa matematica divergerebbero in silenzio (lezione di HDL_PHASE §2.1).
%
%  E' l'UNICA fonte della matematica ACC-IIDM del progetto: la usa sia il blocco SP2
%  `Donatello_ACC_IIDM` sia il plant closed-loop `cf_plant_lib/ACC_IIDM` (che aggiunge solo
%  l'integrazione). Cancello che verifica entrambi: `run_plant_parity` (vs golden Python).
%
%  ⚠️ DA CHIAMARE **UNA VOLTA PER CONTROL-STEP** (DT = 0.1 s): il filtro OU stima a_l da Δv_l/DT.
%     Chiamarla a ogni clock farebbe vedere Δv_l = 0 per 340 campioni su 341 -> a_l ~ 0, in silenzio.
%     Vedi docs/superpowers/specs/2026-07-14-sp2-donatello-acc-iidm-design.md §5.
%
%  NOTA sul path FIXED (SP3): niente LUT e niente Newton-Raphson. HDL Coder genera `sqrt`, `tanh` e
%  `x^4` NATIVAMENTE; la divisione la accetta **solo** con RoundingMethod 'Zero' (con 'Nearest' la
%  rifiuta). `exp` e' l'unica non generabile -- ed e' il motivo per cui la sigmoide richiese una LUT
%  mentre `tanh` no: qui compare solo in ALPHA, che ha argomento COSTANTE e viene ripiegata a
%  build-time. Tutto misurato il 2026-07-15, spec SP3 §2.
  if nargin < 7 || isempty(T), T = acc_types('double'); end
  isFx = ~isa(T.out, 'double');
  DT = 0.1; ALPHA = exp(-DT/1.0); COOL = 0.99;
  % `T_` (time headway IDM) e NON `T`: `T` e' il parametro dei tipi. Ombreggiarlo romperebbe il path
  % fixed, che usa T.st/T.par/T.acc/T.out DOPO questa riga.
  v0 = max(p(1), 1e-3); T_ = max(p(2), 1e-3); s0 = p(3); a = max(p(4), 1e-3); b = max(p(5), 1e-3);

  % Init con guardia `isempty` PER VARIABILE (idioma codegen-safe del progetto, come snn_core.m:15-19):
  % il codegen riconosce letteralmente isempty(<persistent>) come prova di definizione, e senza fallisce
  % con "Persistent variable 'alf' is undefined on some execution paths". `rst` azzera il filtro OU
  % a inizio traiettoria; al primo giro ci pensa gia' isempty, quindi non serve un flag `started`.
  persistent alf vlp
  if isempty(alf) || rst, alf = cast(0, 'like', T.acc);   end
  if isempty(vlp) || rst, vlp = cast(v_l, 'like', T.st); end

  % Niente `setfimath` e niente ramo isFx qui: la fimath ('Zero' per le divisioni) e' gia' nei
  % prototipi di acc_types, quindi ogni cast se la porta dietro e tutto combacia. In DOUBLE questi
  % cast sono no-op -> il riferimento resta bit-identico (lo prova run_plant_parity).
  % NOMI NUOVI (v0f/Tf_/...) e non riassegnazione: `v0 = cast(v0,'like',T.par)` cambierebbe il tipo
  % di v0 (da sfix21_En13, il tipo del decode, a sfix15_En8) e il codegen lo rifiuta -- "Variable
  % types are incompatible". Una variabile non puo' cambiare ne' TIPO ne' FIMATH (HDL_PHASE §9).
  sq = cast(s,  'like', T.st);   vq = cast(v,   'like', T.st);
  dq = cast(dv, 'like', T.st);   lq = cast(v_l, 'like', T.st);
  v0f = cast(v0, 'like', T.par); Tf_ = cast(T_, 'like', T.par); s0f = cast(s0, 'like', T.par);
  af  = cast(a,  'like', T.par); bf  = cast(b,  'like', T.par);

  % stima a_l (filtro OU su differenze finite del leader)
  alf = cast(ALPHA*alf + (1-ALPHA)*acc_div(T, isFx, lq - vlp, DT), 'like', T.acc);
  vlp = cast(lq, 'like', T.st);

  % --- acc_iidm_accel: IIDM base + CAH + blend ACC (verbatim da build_plant_lib:plant_code) ---
  sab = cast(max(sqrt(af*bf), 1e-6), 'like', T.par);
  s_star = cast(s0f + max(vq*Tf_ + acc_div(T, isFx, vq*dq, 2*sab, 1.74, 2.64), 0), 'like', T.st);
  s_safe = cast(max(sq, 2.0), 'like', T.st);
  v_free = cast(af*(1 - min(acc_div(T, isFx, vq, v0f, 8, 45), 10)^4), 'like', T.acc);
  z = cast(min(acc_div(T, isFx, s_star, s_safe, 2, 150), 20), 'like', T.acc);
  below = (vq <= v0f);
  a_z = cast(af*(1 - z^2), 'like', T.acc);
  if z < 1
    if below, a_iidm = cast(v_free*(1 - z^2), 'like', T.acc); else, a_iidm = cast(v_free, 'like', T.acc); end
  else
    if below, a_iidm = cast(a_z, 'like', T.acc); else, a_iidm = cast(v_free + a_z, 'like', T.acc); end
  end
  a_l_bar = cast(min(alf, af), 'like', T.acc);
  a_cah = cast(a_l_bar - acc_div(T, isFx, max(dq,0)^2, 2*s_safe + 1e-6, 4, 300), 'like', T.acc);
  a_cah = cast(min(max(a_cah, -9), af), 'like', T.acc);
  dd = cast(acc_div(T, isFx, a_iidm - a_cah, bf + 1e-6, 0.5, 3), 'like', T.acc);
  a_blend = cast((1-COOL)*a_iidm + COOL*(a_cah + bf*tanh(dd)), 'like', T.acc);
  if a_iidm >= a_cah, ac = a_iidm; else, ac = a_blend; end
  accel = cast(min(max(ac, -9), af), 'like', T.out);

  % [SP4-M-FSM G1] Coppie (num,den) REALI delle 5 divisioni variabili, per il gate di bit-identita' del
  % blocco Divide (probe_divide_bitexact). Ramo nargout-gated: nargout e' coder.const -> il path HDL a 1
  % output (il blocco) NON genera questo ramo, quindi SP3 resta invariato. Cast a T.acc = LOSSLESS: tutti i
  % tipi (st/par/acc/out) hanno f=8 frazionari e T.acc ha il MAX di bit interi (10) -> il valore non cambia
  % (G2 lo ri-verifica sul dataset). Niente double() qui (vietato nel datapath, HDL_PHASE §9): restano fi.
  if nargout >= 2
    pairs = [cast(vq*dq,'like',T.acc),          cast(2*sab,'like',T.acc); ...
             cast(vq,'like',T.acc),             cast(v0f,'like',T.acc); ...
             cast(s_star,'like',T.acc),         cast(s_safe,'like',T.acc); ...
             cast(max(dq,0)^2,'like',T.acc),    cast(2*s_safe + 1e-6,'like',T.acc); ...
             cast(a_iidm - a_cah,'like',T.acc),  cast(bf + 1e-6,'like',T.acc)];
  end
end


function q = acc_div(T, isFx, num, den, lo, hi)
%ACC_DIV  num/den type-parametrica. Fixed: T.recipN==0 -> divide() (SP3); T.recipN>0 -> reciproco-LUT
%  (SP4 var. L) SOLO per divisori VARIABILI (chiamata a 6 arg, con range lo,hi).
%  Un divisore COSTANTE (es. DT nel filtro OU) si chiama a 4 arg (senza lo,hi): resta divide(), che
%  per una costante HDL Coder ripiega in un moltiplicatore shallow -- non e' il problema di profondita'
%  delle 5 divisioni a divisore variabile. `nargin` e' coder.const per specializzazione -> HDL-safe.
  if isFx
    if T.recipN > 0 && nargin >= 6
      q = cast(num * acc_recip_lut(den, lo, hi, T.recipN), 'like', T.acc);
    else
      q = divide(numerictype(T.acc), num, den);
    end
  else
    q = num / den;
  end
end


function T = acc_types(dt, nfrac, recipN)
%ACC_TYPES  Prototipi di tipo per `acc_iidm_open` type-parametrizzato (modello: snn_types.m).
%  dt = 'double' (riferimento algoritmico + plant cf_plant_lib) | 'fixed' (blocco HDL-ready).
%  nfrac (opz.) = bit frazionari del path fixed; i bit INTERI restano FISSI (il range non cambia),
%  varia solo la risoluzione -> e' la manopola dello sweep (run_acc_fixed_sweep), esattamente come
%  snn_types/run_fixed_sweep fanno per la rete.
%
%  I bit INTERI sono dimensionati con DUE criteri diversi, perche' i limiti hanno natura diversa --
%  applicare a tutti la stessa regola sarebbe misurare la cosa sbagliata:
%
%  (A) limitati dall'OSSERVAZIONE -> margine >= 2x sul massimo misurato (il dataset non e' il mondo).
%      Range misurati su 60 traiettorie x 1000 step coi parametri veri stimati dalla rete (spec SP3 §3):
%    st  : s, v, dv, v_l, s_safe, s_star         max misurato  465.77 -> int 10 (|x|<1024, 2.2x)
%    acc : v_free, a_z, a_iidm, a_cah, a_blend,
%          alf, a_l_bar, dd, z, dv^2/(2*s_safe)  min misurato -288.33 -> int 10 (|x|<1024, 3.6x)
%
%  (B) limitati da un CLAMP -> basta che il tipo copra il limite: non e' una stima, non puo' sforare.
%      Un margine di 1.4x su un limite CERTO vale piu' di 2x su un massimo osservato.
%    par : v0,T,s0,a,b   il decode li vincola a [param_lo, param_hi] = [8 .5 1 .3 .5]..[45 2.5 5 2.5 3]
%                        (sigmoide * range + lo: non puo' uscirne)   -> int  6 (|x|<64, 1.4x su 45)
%    out : accel         il codice la clampa a [-9, a], con a <= 2.5 -> int  4 (|x|<16, 1.8x su 9)
  % nfrac di DEFAULT = 8: il MINIMO che rispetta il budget DERIVATO. Misurato da run_acc_fixed_sweep
  % sul dataset INTERO (60 traj x 1000 step = 60.000 campioni, 2026-07-16, log sweep_nfrac8_60traj.log):
  %   budget  E_snn  (footprint in accel della quantizzazione GIA' accettata della rete):
  %                                   p99 = 0.272054   max = 1.48433  [m/s^2]
  %   nfrac=6 E_iidm  p99 = 0.324937  max = 1.78485  -> NON passa (l'IIDM diventerebbe la fonte
  %                                                     d'errore DOMINANTE, scavalcando la rete)
  %   nfrac=8 E_iidm  p99 = 0.156047  max = 0.83368  -> passa, margine ~1.75x su entrambi
  % ⚠️ Passa STRETTO: un dry-run su 2 traiettorie dava ~6x di margine, il dataset intero dice 1.75x.
  %    Le code stanno solo nel campione completo -> non tarare questo numero su pochi casi.
  if nargin < 2, nfrac = 8; end
  % recipN: strategia di divisione del path fixed. 0 = divide() digit-recurrence (SP3, combinatorio
  % profondo). >0 = reciproco a LUT a recipN punti + moltiplica (SP4 variante L). Vive nei tipi cosi'
  % la scelta e' coder.const e single-source. Default 0 = comportamento SP3 invariato.
  if nargin < 3, recipN = 0; end
  switch dt
    case 'double'
      z = double([]);
      T = struct('st', z, 'par', z, 'acc', z, 'out', z);
      T.recipN = 0;
    case 'fixed'
      f = nfrac;
      % La fimath fa parte del TIPO, non e' una decorazione locale. Due ragioni, entrambe misurate:
      %  1) RoundingMethod 'Zero' e' l'UNICA forma di divisione che HDL Coder genera per tipi signed
      %     ('Floor' vale solo per unsigned, 'Nearest' viene rifiutata) -- spec SP3 §2;
      %  2) attaccarla qui evita che una `setfimath` locale la cambi su una variabile gia' assegnata:
      %     il codegen rifiuta anche il cambio di FIMATH, non solo di tipo -- "Properties of fimath
      %     object must match. Property 'RoundMode' is 'nearest' ... but 'fix'". Mettendola nel
      %     prototipo, ogni cast(x,'like',T.*) la porta con se' e tutto combacia per costruzione.
      % Prodotti e somme a precisione FISSA: senza, i word-length crescerebbero a ogni operazione.
      FM = fimath('RoundingMethod', 'Zero', 'OverflowAction', 'Saturate', ...
                  'ProductMode', 'SpecifyPrecision', ...
                  'ProductWordLength', 11 + f, 'ProductFractionLength', f, ...
                  'SumMode', 'SpecifyPrecision', ...
                  'SumWordLength', 11 + f, 'SumFractionLength', f);
      % Prototipi con valore 0 e NON `fi([])`: un campo VUOTO e' "empty-typed" e HDL Coder lo rifiuta
      % quando lo struct dei tipi attraversa piu' funzioni -- "Struct in expression 'acc_types(''fixed'')'
      % has an empty-typed field. This is not supported for MATLAB-to-dataflow conversion" (SP4-M-FSM:
      % le funzioni-fase iidm_prep/nd/use/final). Come PROTOTIPO e' equivalente: `cast(x,'like',T.*)` usa
      % solo numerictype+fimath, che qui sono identici -> nessun cambiamento numerico (lo provano
      % run_plant_parity, run_block_acciidm_test e G2, tutti ri-eseguiti dopo questa modifica).
      T = struct( ...
        'st',  fi(0, true, 11 + f, f, FM), ...   % Q10.f
        'par', fi(0, true,  7 + f, f, FM), ...   % Q6.f
        'acc', fi(0, true, 11 + f, f, FM), ...   % Q10.f
        'out', fi(0, true,  5 + f, f, FM));      % Q4.f
      T.recipN = recipN;
    otherwise
      error('acc_types:dt', 'dt deve essere ''double'' o ''fixed''');
  end
end
